simulink model "slb_logical_opp"  (R2015b)
settings: Solver=FixedStepDiscrete  SolverMode=SingleTasking  StartTime=0.0  StopTime=3  RelTol=1e-3
libraries: simulink x2, hdlsllib x1
settings Model: Creator=at-mt  LastModifiedBy=amatsumo
settings DataIOCC: SaveFormat=Array  SignalLoggingSaveFormat=ModelDataLogs  SaveOutput=off  SignalLogging=off  SaveTime=off
settings OptimizationCC: BlockReduction=off  ConditionallyExecuteInputs=off  DefaultParameterBehavior=Inlined  ExpressionDepthLimit=2147483647
settings DebuggingCC: AlgebraicLoopMsg=error  UnderspecifiedInitializationDetection=Classic  MergeDetectMultiDrivingBlocksExec=none  SolverPrmCheckMsg=warning  SingleTaskRateTransMsg=error  FcnCallInpInsideContextMsg=UseLocalSettings  StateNameClashWarn=warning
settings HardwareCC: ProdBitPerPointer=32  ProdLargestAtomicFloat=None  ProdIntDivRoundTo=Undefined  ProdEndianess=Unspecified  ProdWordSize=32  ProdHWDeviceType=ASIC/FPGA->ASIC/FPGA  ProdEqTarget=off
settings SFSimCC: SFSimEcho=off  SimParseCustomCode=off
settings GRTTargetCC: GeneratePreprocessorConditionals=Disable all  CombineOutputUpdateFcns=off  GRTInterface=on
settings ConfigComp: CovModelRefEnable=Off  CovSFcnEnable=off

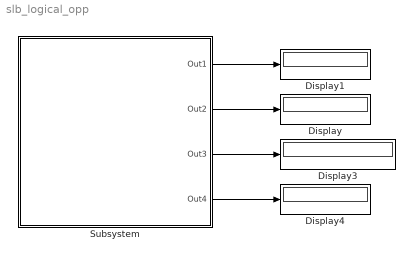
== system slb_logical_opp ==
  Display{,1,3..4} (4 alike) : Display
      Display settings: Format=binary (Stored Integer)
      Display3 settings: Format=binary (Stored Integer)
  Subsystem : Subsystem
  wires:
  Subsystem/2(Out2) -> Display/1
  Subsystem/1(Out1) -> Display1/1
  Subsystem/3(Out3) -> Display3/1
  Subsystem/4(Out4) -> Display4/1

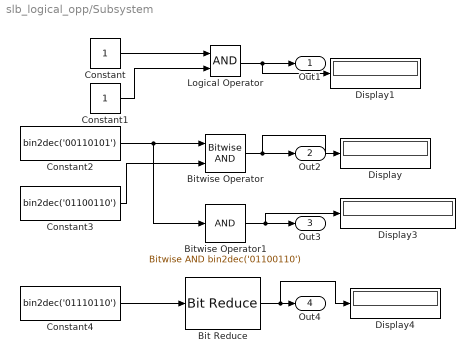
== system slb_logical_opp/Subsystem ==
  Bit Reduce : hdlsllib/HDL Operations/Bit Reduce  mode=XOR
  Bitwise Operator : simulink/Logic and Bit Operations/Bitwise Operator  logicop=AND  UseBitMask=off  NumInputPorts=2  BitMask=bin2dec('11011001')  BitMaskRealWorld=Stored Integer
  Bitwise Operator1 : simulink/Logic and Bit Operations/Bitwise Operator  logicop=AND  UseBitMask=on  BitMask=bin2dec('01100110')  BitMaskRealWorld=Stored Integer
  Constant : Constant  OutDataTypeStr=boolean  SampleTime=1
  Constant1 : Constant  OutDataTypeStr=boolean  SampleTime=1
  Constant2 : Constant  Value=bin2dec('00110101')  OutDataTypeStr=int8  SampleTime=1
  Constant3 : Constant  Value=bin2dec('01100110')  OutDataTypeStr=int8  SampleTime=1
  Constant4 : Constant  Value=bin2dec('01110110')  OutDataTypeStr=int8  SampleTime=1
  Display{,1,3..4} (4 alike) : Display
      settings: Format=binary (Stored Integer)
  Logical Operator : Logic  AllPortsSameDT=off  OutDataTypeStr=boolean
  Out1 : Outport
  Out2 : Outport  Port=2
  Out3 : Outport  Port=3
  Out4 : Outport  Port=4
  wires:
  Constant/1 -> Logical Operator/1
  Constant1/1 -> Logical Operator/2
  Constant2/1 -> Bitwise Operator1/1, Bitwise Operator/1
  Bitwise Operator/1 -> Out2/1, Display/1
  Constant3/1 -> Bitwise Operator/2
  Logical Operator/1 -> Out1/1, Display1/1
  Bitwise Operator1/1 -> Out3/1, Display3/1
  Constant4/1 -> Bit Reduce/1
  Bit Reduce/1 -> Display4/1, Out4/1
